simulink library "TemperatureSomanetChecker"  (R2016b)
settings: Solver=VariableStepAuto  StartTime=0.0  StopTime=10.0  RelTol=1e-3
undefined symbols (not defined in the file): maxTemperatureSomanet
settings Model: Creator=Nathan  LastModifiedBy=RKFE

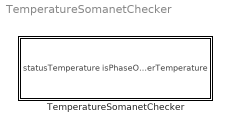
== system TemperatureSomanetChecker ==
  TemperatureSomanetChecker : Subsystem

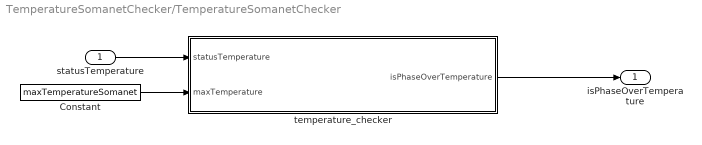
== system TemperatureSomanetChecker/TemperatureSomanetChecker ==
  statusTemperature : Inport  BusOutputAsStruct=on
  Constant : Constant  Value=maxTemperatureSomanet  VectorParams1D=off  SampleTime=-1
  temperature_checker : MATLAB Function  TreatAsAtomicUnit=on
  isPhaseOverTemperature : Outport
  wires:
  statusTemperature/1 -> temperature_checker/1(statusTemperature)
  temperature_checker/1(isPhaseOverTemperature) -> isPhaseOverTemperature/1
  Constant/1 -> temperature_checker/2(maxTemperature)

== matlab function TemperatureSomanetChecker/temperature_checker ==
  data: statusTemperature input; isPhaseOverTemperature output; maxTemperature input
function isPhaseOverTemperature = temperature_checker(statusTemperature,maxTemperature)


if(statusTemperature >= maxTemperature)
    isPhaseOverTemperature = 1;
    %Checks if the measured temperature does not exceed the maximum allowed
    %temperature
    
else
    isPhaseOverTemperature = 0;
end
